simulink model "main"  (R2014b)
settings: Solver=ode3  SolverMode=SingleTasking  StartTime=0.0  StopTime=inf  RelTol=1e-3
libraries: legonxtlib x6
settings Model: SimulationMode=external  CovSFcnEnable=on  ExtModeTrigDuration=2  Creator=Damjan  LastModifiedBy=unixy
settings OptimizationCC: UseDivisionForNetSlopeComputation=off  OptimizeModelRefInitCode=on  LifeSpan=1  SimCompilerOptimization=off
settings DebuggingCC: UnderspecifiedInitializationDetection=Classic  MergeDetectMultiDrivingBlocksExec=none  SolverPrmCheckMsg=none  FrameProcessingCompatibilityMsg=error
settings HardwareCC: ProdLargestAtomicInteger=Long  ProdLargestAtomicFloat=Float  ProdEndianess=LittleEndian  ProdHWDeviceType=ARM Compatible->ARM 7
settings RTWCC: SystemTargetFile=realtime.tlc  GenerateMakefile=off  TemplateMakefile=realtime.tmf  Description=Run on Target Hardware  RTWVerbose=off  RTWCompilerOptimization=off
settings STFCustomTargetCC: TargetLibSuffix=.a  GenerateSampleERTMain=on  ERTCustomFileBanners=on  SupportNonInlinedSFcns=off  SupportVariableSizeSignals=on  MATLABClassNameForMDSCustomization=Simulink.SoftwareTarget.ERTCustomization  GRTInterface=off  SystemTargetFile=realtime.tlc
settings ERTTargetCC: GenerateSampleERTMain=on  ParMdlRefBuildCompliant=off  CompOptLevelCompliant=off  ConcurrentExecutionCompliant=off  CombineOutputUpdateFcns=off  ERTFirstTimeCompliant=off  SupportContinuousTime=on  SupportVariableSizeSignals=on  ModelStepFunctionPrototypeControlCompliant=off  CPPClassGenCompliant=off  ExtModeTransport=2  ExtModeMexFile=ext_serial_win32_comm_no_acks_rtt  ExtModeMexArgs=0 1 9600  InlinedParameterPlacement=NonHierarchical  ERTSrcFileBannerTemplate=realtime_code_template.cgt  ERTHdrFileBannerTemplate=realtime_code_template.cgt  ERTDataSrcFileTemplate=realtime_code_template.cgt  ERTDataHdrFileTemplate=realtime_code_template.cgt  ERTCustomFileTemplate=realtime_file_process.tlc

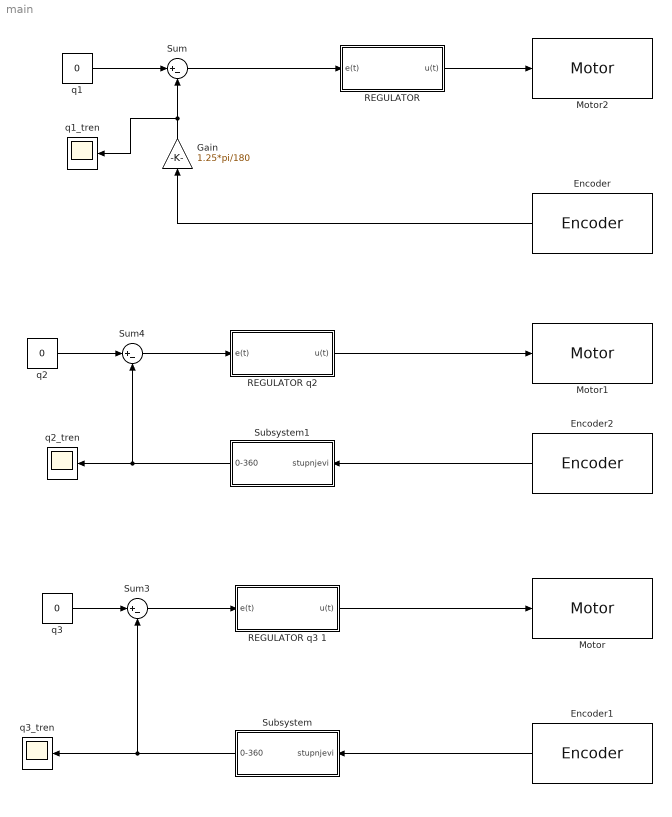
== system main ==
  Encoder : legonxtlib/Encoder  portNumber=C  opMode=No reset  sampleTime=0.1  blockPlatform=LegoMindstormsNXT
  Encoder1 : legonxtlib/Encoder  portNumber=A  opMode=No reset  sampleTime=0.1  blockPlatform=LegoMindstormsNXT
  Encoder2 : legonxtlib/Encoder  portNumber=B  opMode=No reset  sampleTime=0.1  blockPlatform=LegoMindstormsNXT
  Gain : Gain  Gain=1.25*pi/180
  Motor : legonxtlib/Motor  sportNumber=A  sstopAction=Brake  blockPlatform=LegoMindstormsNXT
  Motor1 : legonxtlib/Motor  sportNumber=B  sstopAction=Brake  blockPlatform=LegoMindstormsNXT
  Motor2 : legonxtlib/Motor  sportNumber=C  sstopAction=Brake  blockPlatform=LegoMindstormsNXT
  "REGULATOR " : Subsystem
  REGULATOR q2 : Subsystem
  REGULATOR q3 1 : Subsystem
  Subsystem : Subsystem
  Subsystem1 : Subsystem
  Sum : Sum  Inputs=|+-
  Sum3 : Sum  Inputs=|+-
  Sum4 : Sum  Inputs=|+-
  q1 : Constant  Value=0  SampleTime=1
  q1_tren : Scope
      settings: TimeRange=5  YMin=2  YMax=4.5
  q2 : Constant  Value=0  SampleTime=1
  q2_tren : Scope
      settings: TimeRange=5  YMin=67  YMax=69  SaveName=ScopeData2
  q3 : Constant  Value=0  SampleTime=1
  q3_tren : Scope
      settings: TimeRange=5  YMin=79  YMax=81
  wires:
  Encoder2/1 -> Subsystem1/1(stupnjevi)
  REGULATOR q3 1/1("u(t) ") -> Motor/1
  q3/1 -> Sum3/1
  Sum3/1 -> REGULATOR q3 1/1("e(t) ")
  q2/1 -> Sum4/1
  Sum4/1 -> REGULATOR q2/1("e(t) ")
  REGULATOR q2/1("u(t) ") -> Motor1/1
  Encoder1/1 -> Subsystem/1(stupnjevi)
  Encoder/1 -> Gain/1
  q1/1 -> Sum/1
  Sum/1 -> "REGULATOR "/1("e(t) ")
  "REGULATOR "/1("u(t) ") -> Motor2/1
  Gain/1 -> Sum/2, q1_tren/1
  Subsystem1/1(0-360) -> q2_tren/1, Sum4/2
  Subsystem/1(0-360) -> Sum3/2, q3_tren/1

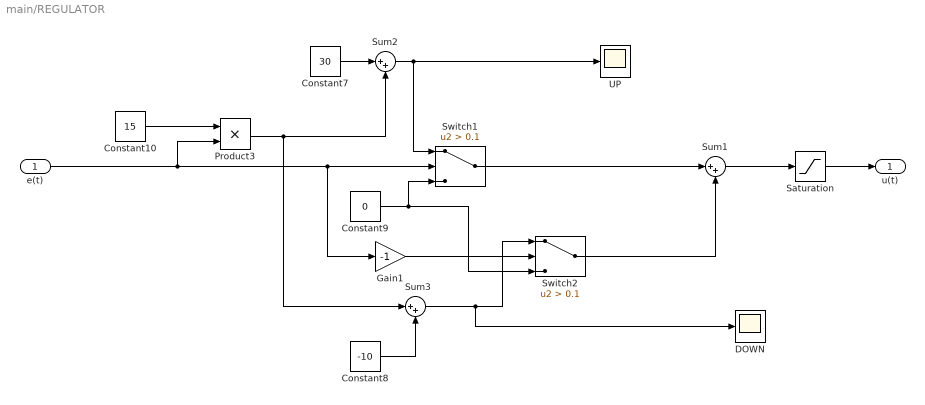
== system main/REGULATOR  ==
  "e(t) " : Inport
  Constant10 : Constant  Value=15
  Constant7 : Constant  Value=30
  Constant8 : Constant  Value=-10
  Constant9 : Constant  Value=0
  DOWN : Scope
      settings: YMin=304  YMax=306  SaveName=ScopeData3
  Gain1 : Gain  Gain=-1
  Product3 : Product
  Saturation : Saturate  UpperLimit=100  LowerLimit=-80
  Sum1 : Sum  Inputs=|++
  Sum2 : Sum  Inputs=|++
  Sum3 : Sum  Inputs=|++
  Switch1 : Switch  Criteria=u2 > Threshold  Threshold=0.1
  Switch2 : Switch  Criteria=u2 > Threshold  Threshold=0.1
  "UP " : Scope
      settings: YMin=304  YMax=306  SaveName=ScopeData4
  "u(t) " : Outport
  wires:
  "e(t) "/1 -> Product3/2, Gain1/1, Switch1/2
  Gain1/1 -> Switch2/2
  Constant9/1 -> Switch2/3, Switch1/3
  Switch2/1 -> Sum1/2
  Switch1/1 -> Sum1/1
  Sum2/1 -> Switch1/1, "UP "/1
  Constant7/1 -> Sum2/1
  Constant10/1 -> Product3/1
  Sum1/1 -> Saturation/1
  Saturation/1 -> "u(t) "/1
  Constant8/1 -> Sum3/2
  Sum3/1 -> DOWN/1, Switch2/1
  Product3/1 -> Sum3/1, Sum2/2

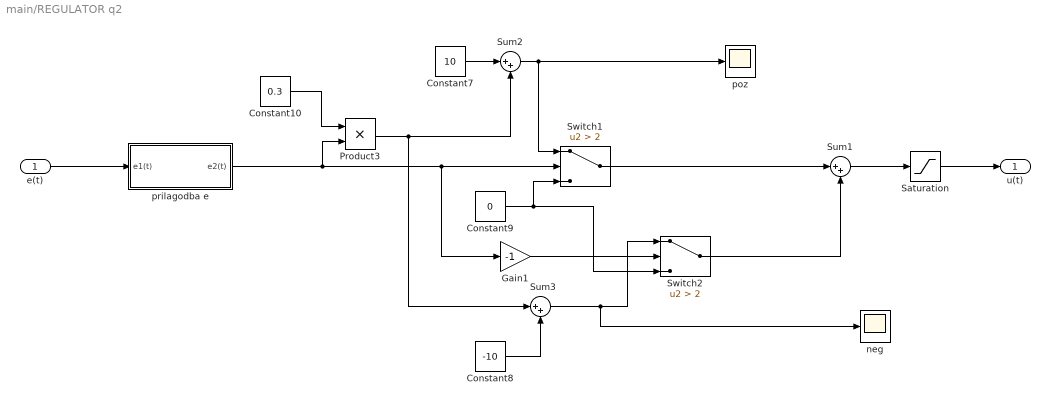
== system main/REGULATOR q2 ==
  "e(t) " : Inport
  Constant10 : Constant  Value=0.3
  Constant7 : Constant  Value=10
  Constant8 : Constant  Value=-10
  Constant9 : Constant  Value=0
  Gain1 : Gain  Gain=-1
  Product3 : Product
  Saturation : Saturate  UpperLimit=100  LowerLimit=-100
  Sum1 : Sum  Inputs=|++
  Sum2 : Sum  Inputs=|++
  Sum3 : Sum  Inputs=|++
  Switch1 : Switch  Criteria=u2 > Threshold  Threshold=2
  Switch2 : Switch  Criteria=u2 > Threshold  Threshold=2
  neg : Scope
      settings: YMin=304  YMax=306  SaveName=ScopeData3
  "poz " : Scope
      settings: YMin=304  YMax=306  SaveName=ScopeData4
  prilagodba e : Subsystem
  "u(t) " : Outport
  wires:
  Gain1/1 -> Switch2/2
  Constant9/1 -> Switch2/3, Switch1/3
  Switch2/1 -> Sum1/2
  Switch1/1 -> Sum1/1
  Sum2/1 -> Switch1/1, "poz "/1
  Constant7/1 -> Sum2/1
  Constant10/1 -> Product3/1
  Constant8/1 -> Sum3/2
  Sum3/1 -> neg/1, Switch2/1
  Product3/1 -> Sum3/1, Sum2/2
  prilagodba e/1(e2(t)) -> Product3/2, Gain1/1, Switch1/2
  "e(t) "/1 -> prilagodba e/1(e1(t))
  Saturation/1 -> "u(t) "/1
  Sum1/1 -> Saturation/1

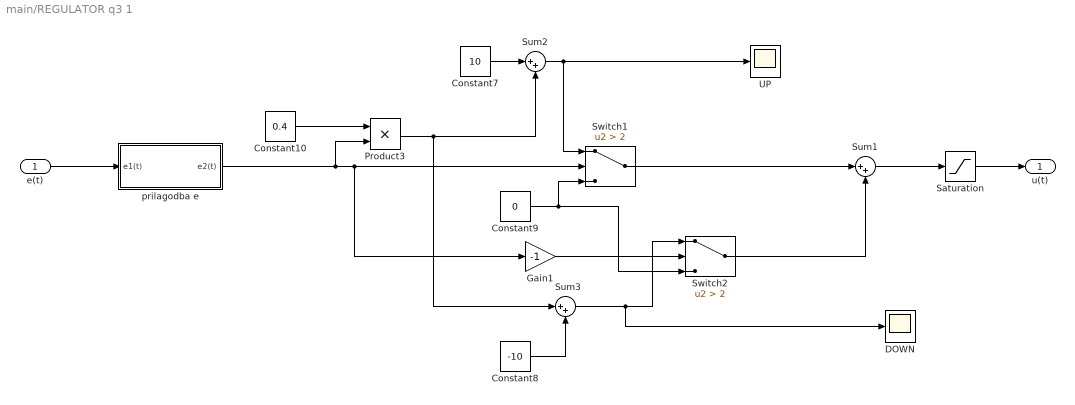
== system main/REGULATOR q3 1 ==
  "e(t) " : Inport
  Constant10 : Constant  Value=0.4
  Constant7 : Constant  Value=10
  Constant8 : Constant  Value=-10
  Constant9 : Constant  Value=0
  DOWN : Scope
      settings: YMin=304  YMax=306  SaveName=ScopeData3
  Gain1 : Gain  Gain=-1
  Product3 : Product
  Saturation : Saturate  UpperLimit=100  LowerLimit=-100
  Sum1 : Sum  Inputs=|++
  Sum2 : Sum  Inputs=|++
  Sum3 : Sum  Inputs=|++
  Switch1 : Switch  Criteria=u2 > Threshold  Threshold=2
  Switch2 : Switch  Criteria=u2 > Threshold  Threshold=2
  "UP " : Scope
      settings: YMin=304  YMax=306  SaveName=ScopeData4
  prilagodba e : Subsystem
  "u(t) " : Outport
  wires:
  Gain1/1 -> Switch2/2
  Constant9/1 -> Switch2/3, Switch1/3
  Switch2/1 -> Sum1/2
  Switch1/1 -> Sum1/1
  Sum2/1 -> Switch1/1, "UP "/1
  Constant7/1 -> Sum2/1
  Constant10/1 -> Product3/1
  Sum1/1 -> Saturation/1
  Saturation/1 -> "u(t) "/1
  Constant8/1 -> Sum3/2
  Sum3/1 -> DOWN/1, Switch2/1
  Product3/1 -> Sum3/1, Sum2/2
  "e(t) "/1 -> prilagodba e/1(e1(t))
  prilagodba e/1(e2(t)) -> Product3/2, Gain1/1, Switch1/2

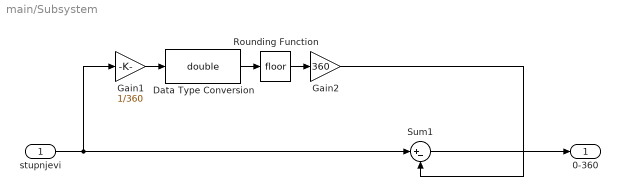
== system main/Subsystem ==
  stupnjevi : Inport
  Data Type Conversion : DataTypeConversion  OutDataTypeStr=double
  Gain1 : Gain  Gain=1/360
  Gain2 : Gain  Gain=360
  Rounding Function : Rounding
  Sum1 : Sum  Inputs=|+-
  0-360 : Outport
  wires:
  stupnjevi/1 -> Sum1/1, Gain1/1
  Rounding Function/1 -> Gain2/1
  Gain2/1 -> Sum1/2
  Gain1/1 -> Data Type Conversion/1
  Data Type Conversion/1 -> Rounding Function/1
  Sum1/1 -> 0-360/1

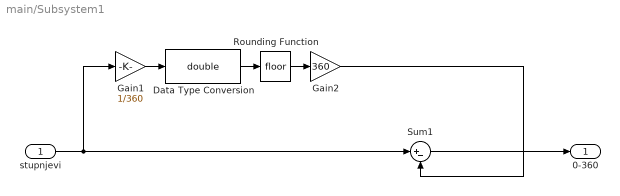
== system main/Subsystem1 ==
  stupnjevi : Inport
  Data Type Conversion : DataTypeConversion  OutDataTypeStr=double
  Gain1 : Gain  Gain=1/360
  Gain2 : Gain  Gain=360
  Rounding Function : Rounding
  Sum1 : Sum  Inputs=|+-
  0-360 : Outport
  wires:
  stupnjevi/1 -> Sum1/1, Gain1/1
  Rounding Function/1 -> Gain2/1
  Gain2/1 -> Sum1/2
  Gain1/1 -> Data Type Conversion/1
  Data Type Conversion/1 -> Rounding Function/1
  Sum1/1 -> 0-360/1

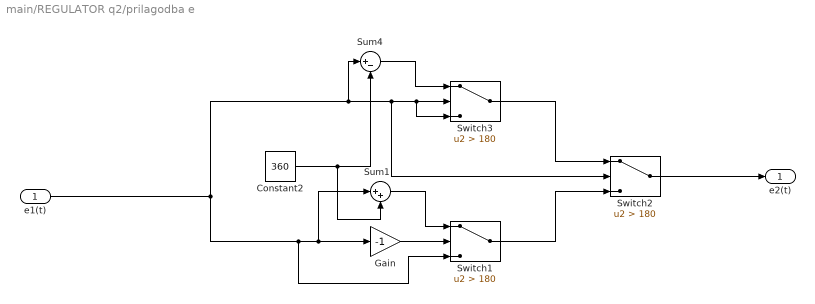
== system main/REGULATOR q2/prilagodba e ==
  e1(t) : Inport
  Constant2 : Constant  Value=360
  Gain : Gain  Gain=-1
  Sum1 : Sum  Inputs=|++
  Sum4 : Sum  Inputs=|+-
  Switch1 : Switch  Criteria=u2 > Threshold  Threshold=180
  Switch2 : Switch  Criteria=u2 > Threshold  Threshold=180
  Switch3 : Switch  Criteria=u2 > Threshold  Threshold=180
  e2(t) : Outport
  wires:
  Switch3/1 -> Switch2/1
  Sum4/1 -> Switch3/1
  Constant2/1 -> Sum4/2, Sum1/2
  Gain/1 -> Switch1/2
  e1(t)/1 -> Sum4/1, Switch2/2, Switch3/3, Switch3/2, Switch1/3, Sum1/1, Gain/1
  Sum1/1 -> Switch1/1
  Switch1/1 -> Switch2/3
  Switch2/1 -> e2(t)/1

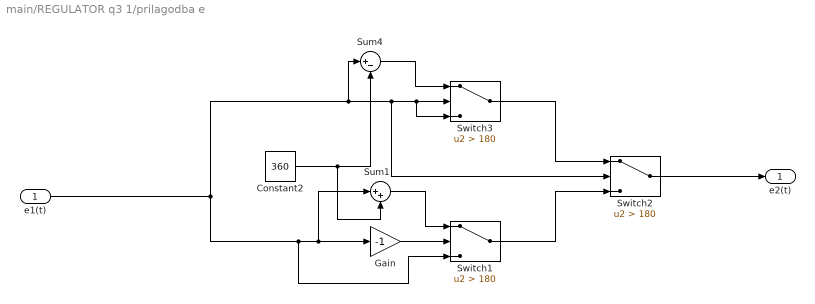
== system main/REGULATOR q3 1/prilagodba e ==
  e1(t) : Inport
  Constant2 : Constant  Value=360
  Gain : Gain  Gain=-1
  Sum1 : Sum  Inputs=|++
  Sum4 : Sum  Inputs=|+-
  Switch1 : Switch  Criteria=u2 > Threshold  Threshold=180
  Switch2 : Switch  Criteria=u2 > Threshold  Threshold=180
  Switch3 : Switch  Criteria=u2 > Threshold  Threshold=180
  e2(t) : Outport
  wires:
  Switch3/1 -> Switch2/1
  Sum4/1 -> Switch3/1
  Constant2/1 -> Sum4/2, Sum1/2
  Gain/1 -> Switch1/2
  e1(t)/1 -> Sum4/1, Switch2/2, Switch3/3, Switch3/2, Switch1/3, Sum1/1, Gain/1
  Sum1/1 -> Switch1/1
  Switch1/1 -> Switch2/3
  Switch2/1 -> e2(t)/1
